simulink model "B_RandomWaterUsage_NoControl"  (R2016a)
settings: Solver=VariableStepAuto  StartTime=0.0  StopTime=10.0  RelTol=1e-3
InitFcn:
  | S1=20;
  | S2=20;
  | h1=5;
  | h2=5;
settings Model: Creator=Hossein  LastModifiedBy=Hossein

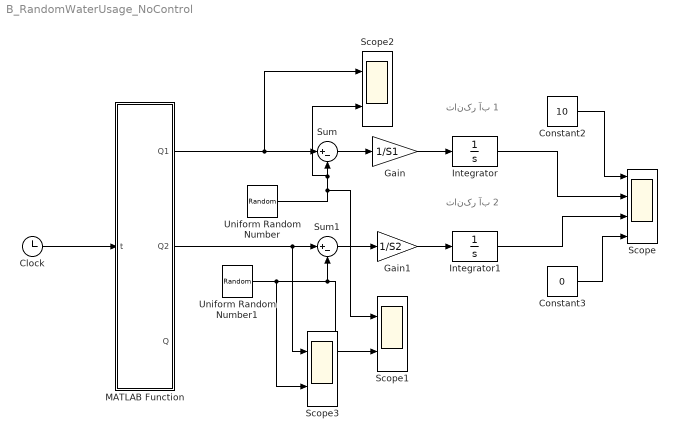
== system B_RandomWaterUsage_NoControl ==
  note: تانکر آب 1
  note: تانکر آب 2
  Clock : Clock
  Constant2 : Constant  Value=10
  Constant3 : Constant  Value=0
  Gain : Gain  Gain=1/S1
  Gain1 : Gain  Gain=1/S2
  Integrator : Integrator  InitialCondition=h1
  Integrator1 : Integrator  InitialCondition=h2
  MATLAB Function : MATLAB Function  TreatAsAtomicUnit=on
  Scope : Scope  NumInputPorts=4
  Scope1 : Scope  NumInputPorts=2
  Scope2 : Scope  NumInputPorts=2
  Scope3 : Scope  NumInputPorts=2
  Sum : Sum  Inputs=|+-
  Sum1 : Sum  Inputs=|+-
  Uniform Random Number : UniformRandomNumber  Minimum=29  Maximum=36  Seed=randi([1,5])  SampleTime=0.4
  Uniform Random Number1 : UniformRandomNumber  Minimum=25  Maximum=33  Seed=randi([1,5])  SampleTime=0.3
  wires:
  Clock/1 -> MATLAB Function/1(t)
  MATLAB Function/1(Q1) -> Scope2/1, Sum/1
  MATLAB Function/2(Q2) -> Scope3/1, Sum1/1
  Sum/1 -> Gain/1
  Gain/1 -> Integrator/1
  Gain1/1 -> Integrator1/1
  Sum1/1 -> Gain1/1
  Integrator/1 -> Scope/2
  Integrator1/1 -> Scope/3
  Constant2/1 -> Scope/1
  Constant3/1 -> Scope/4
  Uniform Random Number/1 -> Scope1/1, Scope2/2, Sum/2
  Uniform Random Number1/1 -> Scope3/2, Scope1/2, Sum1/2

== matlab function B_RandomWaterUsage_NoControl/MATLAB Function ==
  data: t input; Q1 output; Q2 output; Q output
function [Q1,Q2,Q] = fcn(t)
%#codegen

Q1=30;
Q2=30;

Q=Q1+Q2;
